simulink model "obiekt_obserwator_regulator"  (R2016b)
settings: Solver=VariableStepDiscrete  StartTime=0.0  StopTime=5  RelTol=1e-3
values from neighbouring files (symbols this model uses):
  A1 = A.'    [z1.m]
  AL11 = A1(1,1)    [z1.m]
  AL21 = A1(2:3,1)    [z1.m]
  B1 = C.'    [z1.m]
  BL1 = B1(1,1)    [z1.m]
  BL2 = B1(2:3,1)    [z1.m]
  K = acker(A1,B1,p)    [z1.m]
  L = acker(aL1, aL2, pl)    [z1.m]
settings Model: Creator=kamil  LastModifiedBy=kamil

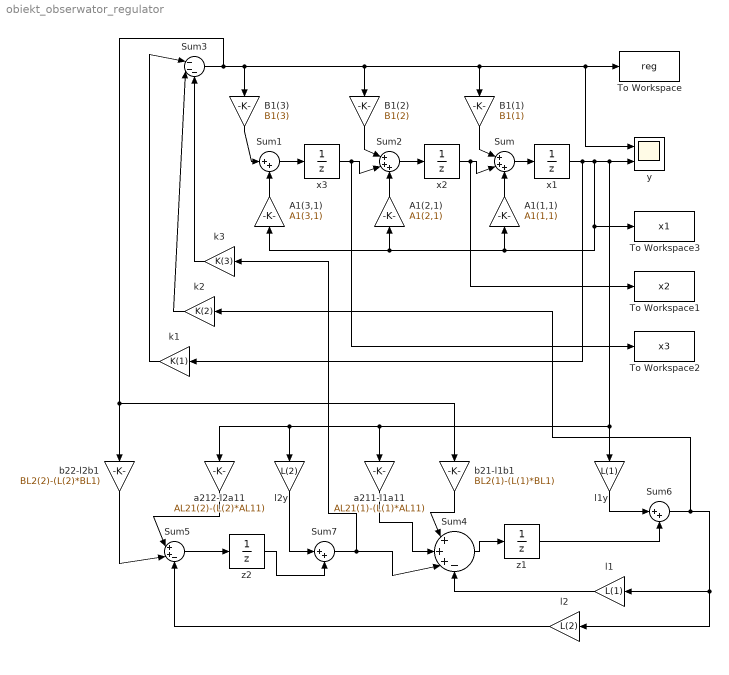
== system obiekt_obserwator_regulator ==
  A1(1,1) : Gain  Gain=A1(1,1)
  A1(2,1) : Gain  Gain=A1(2,1)
  A1(3,1) : Gain  Gain=A1(3,1)
  B1(1) : Gain  Gain=B1(1)
  B1(2) : Gain  Gain=B1(2)
  B1(3) : Gain  Gain=B1(3)
  Sum : Sum  Inputs=|+++
  Sum1 : Sum  Inputs=|++
  Sum2 : Sum  Inputs=|+++
  Sum3 : Sum  Inputs=|---
  Sum4 : Sum  Inputs=|+++-
  Sum5 : Sum  Inputs=|++-
  Sum6 : Sum  Inputs=|++
  Sum7 : Sum  Inputs=|++
  To Workspace : ToWorkspace  VariableName=reg  SaveFormat=Structure With Time  SampleTime=-1
  To Workspace1 : ToWorkspace  VariableName=x2  SaveFormat=Structure With Time  SampleTime=-1
  To Workspace2 : ToWorkspace  VariableName=x3  SaveFormat=Structure With Time  SampleTime=-1
  To Workspace3 : ToWorkspace  VariableName=x1  SaveFormat=Structure With Time  SampleTime=-1
  a211-l1a11 : Gain  Gain=AL21(1)-(L(1)*AL11)
  a212-l2a11 : Gain  Gain=AL21(2)-(L(2)*AL11)
  b21-l1b1 : Gain  Gain=BL2(1)-(L(1)*BL1)
  b22-l2b1 : Gain  Gain=BL2(2)-(L(2)*BL1)
  k1 : Gain  Gain=K(1)
  k2 : Gain  Gain=K(2)
  k3 : Gain  Gain=K(3)
  l1 : Gain  Gain=L(1)
  l1y : Gain  Gain=L(1)
  l2 : Gain  Gain=L(2)
  l2y : Gain  Gain=L(2)
  x1 : UnitDelay  InitialCondition=3  SampleTime=-1
  x2 : UnitDelay  InitialCondition=-1  SampleTime=-1
  x3 : UnitDelay  InitialCondition=1  SampleTime=-1
  y : Scope  NumInputPorts=2
  z1 : UnitDelay  SampleTime=-1
  z2 : UnitDelay  SampleTime=-1
  wires:
  B1(3)/1 -> Sum1/1
  Sum3/1 -> b21-l1b1/1, b22-l2b1/1, y/1, To Workspace/1, B1(1)/1, B1(2)/1, B1(3)/1
  Sum1/1 -> x3/1
  A1(1,1)/1 -> Sum/3
  A1(2,1)/1 -> Sum2/3
  A1(3,1)/1 -> Sum1/2
  Sum/1 -> x1/1
  x2/1 -> To Workspace1/1, Sum/2
  Sum2/1 -> x2/1
  B1(1)/1 -> Sum/1
  B1(2)/1 -> Sum2/1
  k3/1 -> Sum3/3
  k2/1 -> Sum3/2
  k1/1 -> Sum3/1
  x3/1 -> To Workspace2/1, Sum2/2
  z1/1 -> Sum6/2
  Sum4/1 -> z1/1
  Sum5/1 -> z2/1
  l1/1 -> Sum4/4
  l2/1 -> Sum5/3
  l1y/1 -> Sum6/1
  z2/1 -> Sum7/2
  l2y/1 -> Sum7/1
  Sum6/1 -> k2/1, l2/1, l1/1
  Sum7/1 -> k3/1, Sum4/3
  x1/1 -> a211-l1a11/1, a212-l2a11/1, l2y/1, l1y/1, y/2, To Workspace3/1, A1(3,1)/1, A1(2,1)/1, A1(1,1)/1, k1/1
  a212-l2a11/1 -> Sum5/1
  b22-l2b1/1 -> Sum5/2
  a211-l1a11/1 -> Sum4/2
  b21-l1b1/1 -> Sum4/1
